simulink model "estTest_calibration"  (R2021a)
settings: Solver=FixedStepAuto  StartTime=0.0  StopTime=70  FixedStep=0.005  RelTol=1e-3
model workspace (MAT data in the model file):
  Ts = Simulink.Parameter
  Ts.Value = 0.005
  Ts.DataType = 'auto'
  Ts.Dimensions = [1 1]
values from neighbouring files (symbols this model uses):
  Ts = 0.025    [MPCGen_OffsetFree.m]    (also in MPCGen_OffsetFree_UD.m = 0.02; MPCGen_OffsetFree_estDis.m = 0.03; MPCcontrollerGen_OffsetFree.m; MPCcontrollerGen_OffsetFree_UD.m = 0.02)
settings Model: Creator=kboxi  LastModifiedBy=MSI-NB

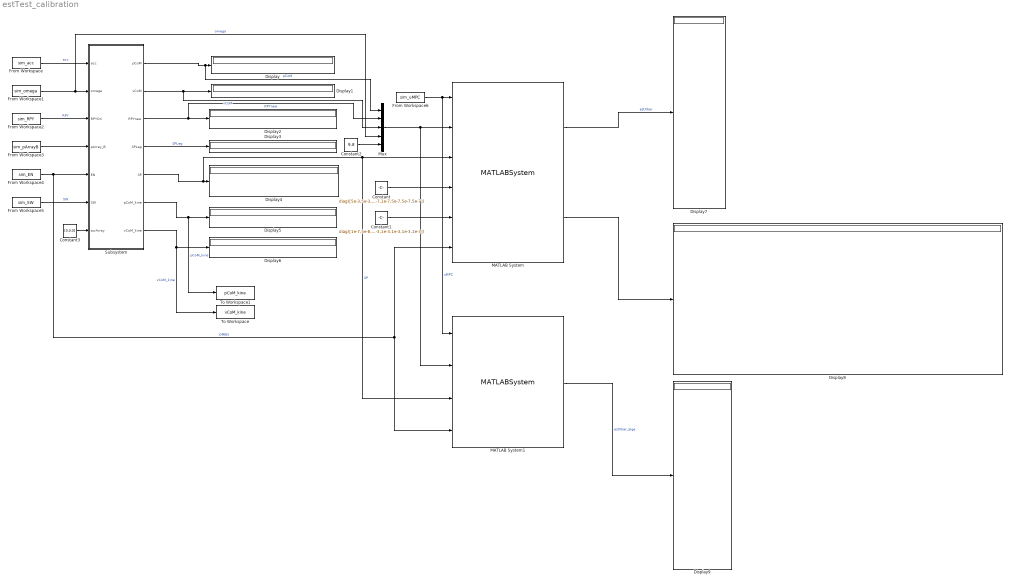
== system estTest_calibration ==
  Constant : Constant  Value=diag([5e-3,5e-3,5e-3,5e-3,5e-3,5e-3,1e-3,1e-3,1e-3,1e-3,1e-3,1e-3,1e-3,1e-7,1e-7,1e-7,5e-7,5e-7,5e-7,1e-7,1e-7,1e-7,5e-7,5e-7,5e-7])
  Constant1 : Constant  Value=diag([1e-7,5e-8,1e-8,1e-6,1e-6,1e-6,1e-5,1e-3,1e-3,1e-3,1e-3,1e-3,1e-3])
  Constant2 : Constant  Value=9.8
  Constant3 : Constant  Value=[0,0,0]
  Display{,1..9} (10 alike) : Display
  From Workspace : FromWorkspace  VariableName=sim_acc  SampleTime=Ts
  From Workspace1 : FromWorkspace  VariableName=sim_omega  SampleTime=Ts
  From Workspace2 : FromWorkspace  VariableName=sim_RPY  SampleTime=Ts
  From Workspace3 : FromWorkspace  VariableName=sim_pArrayB  SampleTime=Ts
  From Workspace4 : FromWorkspace  VariableName=sim_EN  SampleTime=Ts
  From Workspace5 : FromWorkspace  VariableName=sim_SW  SampleTime=Ts
  From Workspace6 : FromWorkspace  VariableName=sim_uMPC  SampleTime=Ts
  MATLAB System : MATLABSystem  System=KalmanFilter_DIY_MPCDis  Ts=0.005  m=3  Inorm=diag( [0.0046125 0.0230942 0.0253262] )  SimulateUsing=Code generation
      mask Type: KalmanFilter_DIY_MPCDis
      mask Display:
      | disp('KalmanFilter_DIY_MPCDis');
      | port_label('input',1,'U_MPC');
      | port_label('input',2,'xFB');
      | port_label('input',3,'pW');
      | port_label('input',4,'Q');
      | port_label('input',5,'R');
      | port_label('input',6,'Reset');
      | port_label('output',1,'estXbar');
      | port_label('output',2,'P');
  MATLAB System1 : MATLABSystem  System=algebraicDisEstmator  Ts=0.005  m=3  Inorm=diag( [0.0046125 0.0230942 0.0253262] )  SimulateUsing=Code generation
      mask Type: algebraicDisEstmator
      mask Display:
      | disp('algebraicDisEstmator');
      | port_label('input',1,'U_MPC');
      | port_label('input',2,'xFB');
      | port_label('input',3,'pW');
      | port_label('input',4,'Reset');
      | port_label('output',1,'estXbar');
  Mux : Mux  Inputs=5
  Subsystem : Subsystem
  To Workspace : ToWorkspace  VariableName=vCoM_kine  SaveFormat=Structure With Time  SampleTime=-1
  To Workspace1 : ToWorkspace  VariableName=pCoM_kine  SaveFormat=Structure With Time  SampleTime=-1
  wires:
  From Workspace3/1 -> Subsystem/4(pArray_B)
  Subsystem/3(RPYnew) -> Mux/2, Display2/1  "RPYnew"
  From Workspace2/1 -> Subsystem/3(RPYOri)  "RPY"
  Subsystem/5(SP) -> MATLAB System1/3, MATLAB System/3, Display4/1  "SP"
  Subsystem/2(vCoM) -> Mux/3, Display1/1  "vCoM"
  Constant3/1 -> Subsystem/7(surArray)
  Subsystem/4(SPLeg) -> Display3/1  "SPLeg"
  Subsystem/1(pCoM) -> Mux/1, Display/1  "pCoM"
  From Workspace5/1 -> Subsystem/6(SW)  "SW"
  From Workspace/1 -> Subsystem/1(acc)  "acc"
  From Workspace1/1 -> Subsystem/2(omega), Mux/4  "omega"
  From Workspace4/1 -> Subsystem/5(EN), MATLAB System/6, MATLAB System1/4  "OffEN"
  Subsystem/6(pCoM_kine) -> To Workspace1/1, Display5/1  "pCoM_kine"
  Subsystem/7(vCoM_kine) -> To Workspace/1, Display6/1  "vCoM_kine"
  Mux/1 -> MATLAB System1/2, MATLAB System/2
  MATLAB System/1 -> Display7/1  "estXbar"
  Constant/1 -> MATLAB System/4
  Constant1/1 -> MATLAB System/5
  Constant2/1 -> Mux/5
  From Workspace6/1 -> MATLAB System1/1, MATLAB System/1  "uMPC"
  MATLAB System/2 -> Display8/1
  MATLAB System1/1 -> Display9/1  "estXbar_alge"

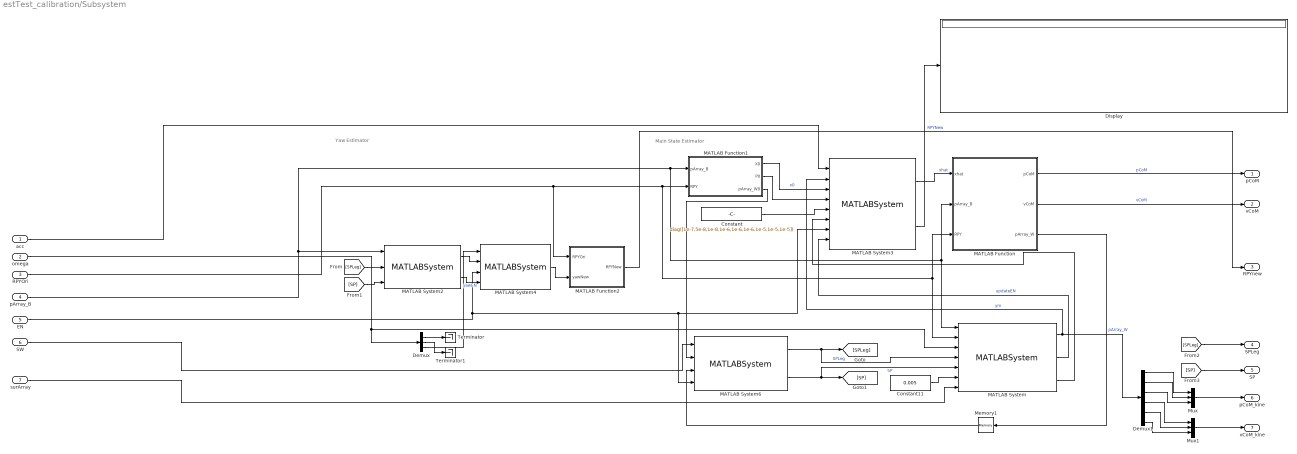
== system estTest_calibration/Subsystem ==
  note: Yaw Estimator
  note: Main State Estimator
  acc : Inport
  omega : Inport  Port=2
  RPYOri : Inport  Port=3
  pArray_B : Inport  Port=4
  EN : Inport  Port=5
  SW : Inport  Port=6
  surArray : Inport  Port=7
  Constant : Constant  Value=diag([1e-7,5e-8,1e-8,1e-6,1e-6,1e-6,1e-5,1e-5,1e-5])
  Constant11 : Constant  Value=0.005
  Demux : Demux  Outputs=3
  Demux1 : Demux  Outputs=6
  Display : Display
  MATLAB Function : MATLAB Function  TreatAsAtomicUnit=on
  MATLAB Function1 : MATLAB Function  TreatAsAtomicUnit=on
  MATLAB Function2 : MATLAB Function  TreatAsAtomicUnit=on
  MATLAB System : MATLABSystem  System=estX_byJoint  SimulateUsing=Code generation
      mask Type: estX_byJoint
      mask Display:
      | disp('estX_byJoint');
      | port_label('input',1,'pArray_B');
      | port_label('input',2,'RPY');
      | port_label('input',3,'omegaB');
      | port_label('input',4,'SPLeg');
      | port_label('input',5,'SP');
      | port_label('input',6,'dt');
      | port_label('input',7,'surPara');
      | port_label('output',1,'ym');
      | port_label('output',2,'updateEN');
      | port_label('output',3,'KF_R');
  MATLAB System2 : MATLABSystem  System=yawEst_byJoint  dt=0.005  SimulateUsing=Code generation
      mask Type: yawEst_byJoint
      mask Display:
      | disp('yawEst_byJoint');
      | port_label('input',1,'pArray_B');
      | port_label('input',2,'SPLeg');
      | port_label('input',3,'SP');
      | port_label('output',1,'yawKine');
      | port_label('output',2,'updateEN');
  MATLAB System3 : MATLABSystem  System=KalmanFilter_DIY_Offrm  Ts=0.005  SimulateUsing=Code generation
      mask Type: KalmanFilter_DIY_Offrm
      mask Display:
      | disp('KalmanFilter_DIY_Offrm');
      | port_label('input',1,'u');
      | port_label('input',2,'y');
      | port_label('input',3,'x0');
      | port_label('input',4,'p0');
      | port_label('input',5,'Q');
      | port_label('input',6,'R');
      | port_label('input',7,'Reset');
      | port_label('input',8,'updateEN');
      | port_label('output',1,'xhat');
      | port_label('output',2,'P');
  MATLAB System4 : MATLABSystem  System=KalmanFilter_DIY_yaw  A=1  B=Ts  C=1  G=1  x0=0  p0=1  Q=0.1  R=0.1  SimulateUsing=Code generation
      mask Type: KalmanFilter_DIY_yaw
      mask Display:
      | disp('KalmanFilter_DIY_yaw');
      | port_label('input',1,'u');
      | port_label('input',2,'y');
      | port_label('input',3,'Reset');
      | port_label('input',4,'updateEN');
      | port_label('output',1,'xhat');
  MATLAB System6 : MATLABSystem  System=LegStateIndicator  SimulateUsing=Code generation
      mask Type: LegStateIndicator
      mask Display:
      | disp('LegStateIndicator');
      | port_label('input',1,'SW');
      | port_label('input',2,'pArray_W0');
      | port_label('input',3,'pArray_W');
      | port_label('input',4,'reset');
      | port_label('output',1,'SPLeg');
      | port_label('output',2,'SP');
  Memory1 : Memory  InitialCondition=zeros(12,1)  InheritSampleTime=on
  Mux : Mux  Inputs=3
  Mux1 : Mux  Inputs=3
  Terminator : Terminator
  Terminator1 : Terminator
  pCoM : Outport
  vCoM : Outport  Port=2
  RPYnew : Outport  Port=3
  SPLeg : Outport  Port=4
  SP : Outport  Port=5
  pCoM_kine : Outport  Port=6
  vCoM_kine : Outport  Port=7
  wires:
  Demux/1 -> Terminator/1
  MATLAB System6/2 -> [SP], MATLAB System/5  "SP"
  MATLAB System/1 -> MATLAB System3/2, Demux1/1  "ym"
  MATLAB System/2 -> MATLAB System3/8  "updateEN"
  Demux/3 -> MATLAB System4/1
  [SPLeg] -> MATLAB System2/2
  Constant/1 -> MATLAB System3/5
  MATLAB System4/1 -> MATLAB Function2/2(yawNew)
  MATLAB System2/1 -> MATLAB System4/2
  MATLAB System3/1 -> MATLAB Function/1(xhat)  "xhat"
  pArray_B/1 -> MATLAB System2/1, MATLAB Function1/1(pArray_B), MATLAB Function/2(pArray_B), MATLAB System/1
  MATLAB Function1/1(X0) -> MATLAB System3/3  "x0"
  MATLAB Function/1(pCoM) -> pCoM/1  "pCoM"
  MATLAB System/3 -> MATLAB System3/6
  MATLAB System6/1 -> MATLAB System/4, [SPLeg]  "SPLeg"
  MATLAB Function1/3(pArray_W0) -> MATLAB System6/2
  Demux/2 -> Terminator1/1
  RPYOri/1 -> MATLAB Function2/1(RPYOri), MATLAB Function1/2(RPY), MATLAB Function/3(RPY), MATLAB System/2
  MATLAB Function/2(vCoM) -> vCoM/1  "vCoM"
  EN/1 -> MATLAB System4/3, MATLAB System3/7, MATLAB System6/4
  Constant11/1 -> MATLAB System/6
  MATLAB Function1/2(P0) -> MATLAB System3/4
  surArray/1 -> MATLAB System/7
  MATLAB Function/3(pArray_W) -> Memory1/1  "pArray_W"
  omega/1 -> Demux/1, MATLAB System/3
  MATLAB System2/2 -> MATLAB System4/4  "yawEN"
  [SP] -> MATLAB System2/3
  Memory1/1 -> MATLAB System6/3
  [SPLeg] -> SPLeg/1
  [SP] -> SP/1
  acc/1 -> MATLAB System3/1
  SW/1 -> MATLAB System6/1
  MATLAB Function2/1(RPYNew) -> RPYnew/1  "RPYNew"
  Demux1/1 -> Mux/1
  Demux1/2 -> Mux/2
  Demux1/3 -> Mux/3
  Demux1/4 -> Mux1/1
  Demux1/5 -> Mux1/2
  Demux1/6 -> Mux1/3
  Mux/1 -> pCoM_kine/1
  Mux1/1 -> vCoM_kine/1
  MATLAB System3/2 -> Display/1

== matlab function estTest_calibration/Subsystem/MATLAB Function1 ==
  data: pArray_B input; RPY input; X0 output; P0 output; pArray_W0 output
function [X0,P0,pArray_W0]=fcn(pArray_B,RPY)
% NOTE: pArray_W0 is calculated without the value of yaw angle!!!
Ry=[cos(RPY(2)),0,sin(RPY(2));
    0,1,0;
    -sin(RPY(2)),0,cos(RPY(2))];
Rx=[1,0,0;
    0,cos(RPY(1)),-sin(RPY(1));
    0,sin(RPY(1)),cos(RPY(1))];
pArray_B=reshape(pArray_B,3,4)/1000;
pArray_float=Ry*Rx*pArray_B; % foot-end position in floating coordinate
zOff=-min(pArray_float(3,:));
temp=pArray_float+[0;0;zOff]*[1,1,1,1];
pCoM=[0;0;zOff];
vCoM=[0;0;0];
pArray_W0=[temp(:,1);temp(:,2);temp(:,3);temp(:,4)];
X0=[pCoM;vCoM;zeros(3,1)];
P0=eye(9)*10^-3;

== matlab function estTest_calibration/Subsystem/MATLAB Function ==
  data: xhat input size=[9,1]; pCoM output size=[3,1]; vCoM output size=[3,1]; pArray_B input; RPY input; pArray_W output
function [pCoM,vCoM,pArray_W] = fcn(xhat,pArray_B,RPY)
% pB the CoM position in the world coordinate
% vB the CoM velocity
% Wpi the foot-end position in the world coordinate
pCoM=[xhat(1);xhat(2);xhat(3)];
vCoM=[xhat(4);xhat(5);xhat(6)];
Rz=[cos(RPY(3)),-sin(RPY(3)),0;
    sin(RPY(3)),cos(RPY(3)),0;
    0,0,1];
Ry=[cos(RPY(2)),0,sin(RPY(2));
    0,1,0;
    -sin(RPY(2)),0,cos(RPY(2))];
Rx=[1,0,0;
    0,cos(RPY(1)),-sin(RPY(1));
    0,sin(RPY(1)),cos(RPY(1))];
R=Rz*Ry*Rx;
pArray_B=reshape(pArray_B,3,4)/1000;
temp=R*pArray_B+pCoM*[1,1,1,1];
pArray_W=[temp(:,1);temp(:,2);temp(:,3);temp(:,4)];

== matlab function estTest_calibration/Subsystem/MATLAB Function2 ==
  data: RPYOri input; RPYNew output size=[3 1]; yawNew input
function RPYNew = fcn(RPYOri,yawNew)
RPYNew=zeros(3,1);
RPYNew(1)=RPYOri(1);
RPYNew(2)=RPYOri(2);
RPYNew(3)=yawNew;
